simulink library "seesaw_hw_lib"  (R2026a)
settings: Solver=VariableStepAuto
undefined symbols (not defined in the file): d_select, step_time, ud_neg, ud_pos, V_sat
settings Model: Creator=Karim Negm  LastModifiedBy=Karim Negm

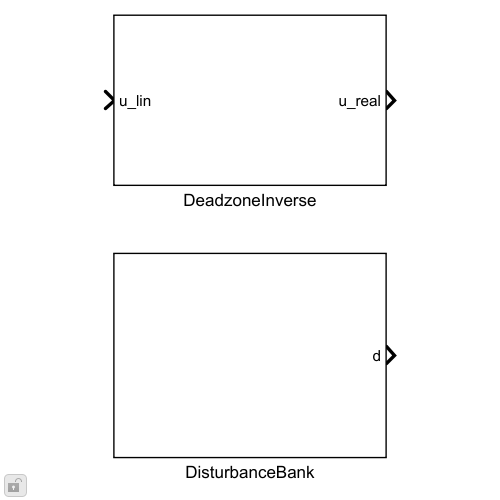
[thumbnail: Simulink's stored preview of the top-level diagram]
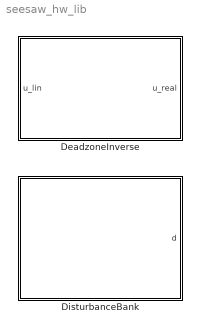
== system seesaw_hw_lib ==
  DeadzoneInverse : Subsystem
  DisturbanceBank : Subsystem

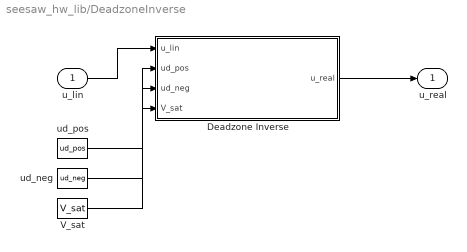
== system seesaw_hw_lib/DeadzoneInverse ==
  u_lin : Inport
  Deadzone Inverse : MATLAB Function  TreatAsAtomicUnit=on
  V_sat : Constant  Value=V_sat
  ud_neg : Constant  Value=ud_neg
  ud_pos : Constant  Value=ud_pos
  u_real : Outport
  wires:
  u_lin/1 -> Deadzone Inverse/1(u_lin)
  ud_pos/1 -> Deadzone Inverse/2(ud_pos)
  ud_neg/1 -> Deadzone Inverse/3(ud_neg)
  V_sat/1 -> Deadzone Inverse/4(V_sat)
  Deadzone Inverse/1(u_real) -> u_real/1

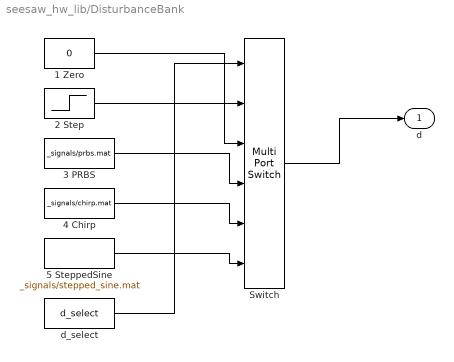
== system seesaw_hw_lib/DisturbanceBank ==
  1 Zero : Constant  Value=0
  2 Step : Step  Time=step_time  FinalValue=step_amp
  3 PRBS : FromFile  FileName=_signals/prbs.mat
  4 Chirp : FromFile  FileName=_signals/chirp.mat
  5 SteppedSine : FromFile  FileName=_signals/stepped_sine.mat
  Switch : MultiPortSwitch  Inputs=5
  d_select : Constant  Value=d_select
  d : Outport
  wires:
  d_select/1 -> Switch/1
  1 Zero/1 -> Switch/2
  2 Step/1 -> Switch/3
  3 PRBS/1 -> Switch/4
  4 Chirp/1 -> Switch/5
  5 SteppedSine/1 -> Switch/6
  Switch/1 -> d/1

== matlab function seesaw_hw_lib/DeadzoneInverse/Deadzone Inverse ==
  data: u_lin input; u_real output; ud_pos input; ud_neg input; V_sat input
function u_real = deadzone_inverse(u_lin, ud_pos, ud_neg, V_sat)
%#codegen
% Replicates PID_seesaw/Non-linear Motor: adds the static-friction
% bias the motor needs to start moving, then clamps to the rail.
epsilon = 0.1;
if u_lin >  epsilon
    u_real = u_lin + ud_pos;
elseif u_lin < -epsilon
    u_real = u_lin - ud_neg;
else
    u_real = 0;
end
if u_real >  V_sat, u_real =  V_sat; end
if u_real < -V_sat, u_real = -V_sat; end
